simulink model "GFLI_full_standard"  (R2024b)
settings: Solver=FixedStepAuto  StartTime=0.0  StopTime=1  FixedStep=Ts  RelTol=1e-3
PreLoadFcn:
  | % Ts = 1e-6;
  | % Ts_Control = 50e-6;
  | %
  | % vlink = 700;
  | % Lf = 2.2e-3;
  | % Cf = 10e-6;
InitFcn:
  | clear all
  | clc
  | %% System parameters
  | Prated = 5e3; %5kW
  | Vg  = 220;     % rms grid voltage
  | Irms = Prated/(sqrt(3)*220*sqrt(3));
  | Ipk = Irms*sqrt(2);
  | 
  | Vdc = 700;     %dc-voltage
  | w1  = 100*pi;   % angular freq
  | fs  = 20e3;
  | Ts = 1/fs;      % control sampling time
  | fsw = 10e3;     % switching freq
  | Tsw = 1/fsw;
  | % grid param
  | Rg = 3e-4;
  | Lg = 1e-3;
  | %% LCL design
  | % Step A — pick inverter-side inductor L1 from ripple 20% Ipk
  | deltaI = 0.02*Ipk;
  | Lf1 = Vdc/(12*fsw*deltaI);
  | Rf1 = 3e-4;
  | % Step B — choose capacitor Cf by limiting reactive power at 50 Hz| Q =
  | %3*Vrms^2*w*Cf| limit ~3% => <= 150Var
  | Cf  = 150/(3*Vg^2*w1);
  | % Step C — choose grid-side inductor| L2/L1 ~ 0.3-1
  | Rf2 = 3e-4;
  | Lf2 = 1.5e-3;
  | % Step D — check resonance frequency|Rule of thumb: 10f1 < fr < 0.5fsw​
  | fr = (1/(2*pi))*sqrt((Lf1+Lf2)/(Lf1*Lf2*Cf));
  | wr = 2*pi*fr;
  | % Step E — damping: Passive damping resistor in series with Cf|
  | rd = 1/(3*wr*Cf);
  | 
  | %% PLL design| Bandwidth choice Typical 10–30 Hz. Choose 20 Hz:
  | wnPll = 2*pi*50;
  | xipll = 0.707;
  | Kp_pll = 2*xipll*wnPll;
  | Ki_pll = wnPll^2;
  | 
  | %% PI current controller|
  | Tresc=0.5e-3;
  | e=1;
  | omega=2*pi/Tresc;
  | k=1/(Lf1+Lf2);
  | Kp_PI=2*e*omega/k;
  | Ki_PI=omega^2/k;
undefined symbols (not defined in the file or in its folder): DiscIntNeverNeededParam, initial
libraries: spsVoltageMeasurementLib x13, spsCurrentMeasurementLib x6, spsIGBTDiodeLib x6, spsSeriesRLCBranchLib x6, powerlib_extras x4, spsThreePhaseSeriesRLCBranchLib x3, spsPLL3phLib x1, spsPWMGenerator2LevelLib x1, spsDCVoltageSourceLib x1, spsThreePhaseSourceLib x1, sps_lib x1
settings Model: Creator=hjyoo  LastModifiedBy=ACER
settings RTWCC: GPUComputeCapability=3.5

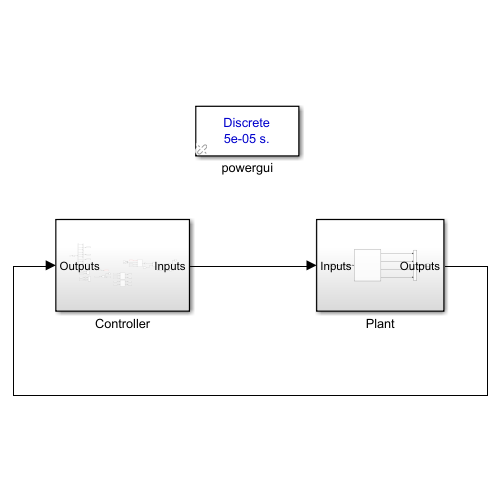
[thumbnail: Simulink's stored preview of the top-level diagram]
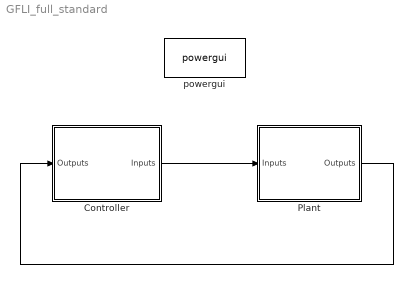
== system GFLI_full_standard ==
  Controller : Subsystem
  Plant : Subsystem
  powergui : sps_lib/powergui  Priority=1  SimulationMode=Discrete  SampleTime=Ts  frequency=60  Iterations=50  frequencyindice=0  Pbase=100e6  ErrMax=1e-4  UnitsV=kV  UnitsW=MW  buscounter=0  FunctionMessages=off  echomessages=off  EnableUseOfTLC=off  CurrentSourceSwitches=off  DisableSnubberDevices=off  DisableRonSwitches=off  DisableVfSwitches=off  DisplayEquations=off  AutomaticDiscreteSolvers=off  SolverType=Tustin/Backward Euler (TBE)  Interpol=off  ExternalGateDelay=off  methode=off  Ts=100  x0status=blocks  SPID=on  SwTol=0  HookPort=off  NonlinearTolerance=1e-4  nMaxIteration=100  ContinueOnMaxIteration=off  RestoreLinks=warning  ResistiveCurrentMeasurement=off  Frange=[0:2:500]  Ylog=off  Xlog=on  ShowGrid=off  save=off  variable=ZData  structure=0  ZoomFFT=off  StartTime=0.0  cycles=1  DisplayStyle=1  fundamental=60  FreqAxis=off  MaxFrequency=1000  frequencyindicesteady=1  RmsSteady=1  display=off
  wires:
  Controller/1(Inputs) -> Plant/1(Inputs)
  Plant/1(Outputs) -> Controller/1(Outputs)

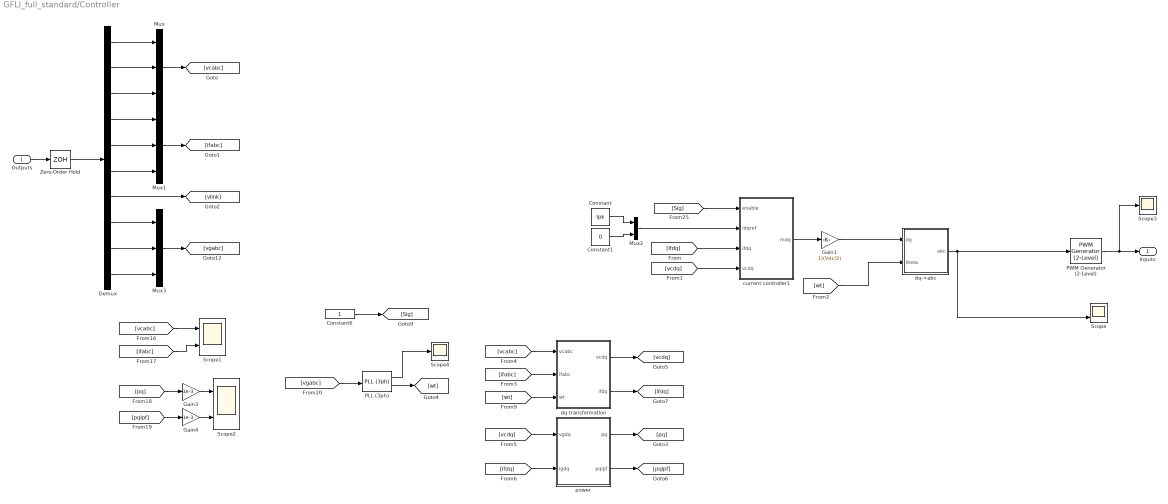
== system GFLI_full_standard/Controller ==
  Outputs : Inport
  Constant : Constant  Value=Ipk
  Constant1 : Constant  Value=0
  Constant6 : Constant
  Demux : Demux  Outputs=10
  Gain1 : Gain  Gain=1/(Vdc/2)
  Gain3 : Gain  Gain=1e-3
  Gain4 : Gain  Gain=1e-3
  Mux : Mux  Inputs=3
  Mux1 : Mux  Inputs=3
  Mux2 : Mux  Inputs=2
  Mux3 : Mux  Inputs=3
  PLL (3ph) : spsPLL3phLib/PLL (3ph)  Fmin=45  Par_Init=[0, 50]  ParK=[180, 3200, 1]  TcD=1e-4  MaxRateChangeFreq=12  FilterCutOffFreq=25  Ts=0  AGC=on
  PWM Generator (2-Level) : spsPWMGenerator2LevelLib/PWM Generator (2-Level)  ModulatorType=Three-phase bridge (6 pulses)  ModulatorMode=Unsynchronized  Fc=fsw  Pc=0  nF=27  MinMax="[ -1  1 ]"  SamplingTechnique=Natural  ModulatingSignals=off  m=0.8  Freq=60  Phase=0  Ts=Ts  ShowCarrierOutport=off
  Scope : Scope  NumInputPorts=2
  Scope1 : Scope  NumInputPorts=2
  Scope2 : Scope  NumInputPorts=2
  Scope3 : Scope
  Scope4 : Scope
  Zero-Order Hold : ZeroOrderHold  SampleTime=Ts
  current controller1 : Subsystem  mask{kp=Kp_PI, ki=Ki_PI, limit=inf, L=Lf1+Lf2, ts=Ts}
      mask prompts: kp "proportional(kp)"; ki "integral(ki)"; limit "saturation limit"; L "inductance(H)"; ts "Sampling Time"
  dq transformation : Subsystem
  dq->abc : Subsystem
  power : Subsystem
  Inputs : Outport
  wires:
  Outputs/1 -> Zero-Order Hold/1
  Demux/1 -> Mux/1
  Demux/2 -> Mux/2
  Demux/3 -> Mux/3
  Demux/5 -> Mux1/2
  Demux/4 -> Mux1/1
  Demux/6 -> Mux1/3
  Mux1/1 -> [ifabc]
  Demux/7 -> [vlink]
  Zero-Order Hold/1 -> Demux/1
  PWM Generator (2-Level)/1 -> Scope3/1, Inputs/1
  Mux/1 -> [vcabc]
  dq transformation/2(ifdq) -> [ifdq]
  dq transformation/1(vcdq) -> [vcdq]
  [vcabc] -> dq transformation/1(vcabc)
  [wt] -> dq transformation/3(wt)
  [ifabc] -> dq transformation/2(ifabc)
  [ifdq] -> current controller1/3(ifdq)
  [wt] -> dq->abc/2(theta)
  dq->abc/1(abc) -> Scope/2, PWM Generator (2-Level)/1
  [vcdq] -> power/1(vgdq)
  power/1(pq) -> [pq]
  [ifdq] -> power/2(igdq)
  power/2(pqlpf) -> [pqlpf]
  [vcdq] -> current controller1/4(vcdq)
  current controller1/1(mdq) -> Gain1/1
  [Sig] -> current controller1/1(enable)
  Constant6/1 -> [Sig]
  [vcabc] -> Scope1/1
  [ifabc] -> Scope1/2
  [pq] -> Gain3/1
  [pqlpf] -> Gain4/1
  Gain3/1 -> Scope2/1
  Gain4/1 -> Scope2/2
  Constant/1 -> Mux2/1
  Constant1/1 -> Mux2/2
  Mux2/1 -> current controller1/2(idqref)
  Mux3/1 -> [vgabc]
  Demux/10 -> Mux3/3
  Demux/8 -> Mux3/1
  Demux/9 -> Mux3/2
  [vgabc] -> PLL (3ph)/1
  PLL (3ph)/2 -> [wt]
  PLL (3ph)/1 -> Scope4/1
  Gain1/1 -> dq->abc/1(dq)

== system GFLI_full_standard/Plant ==
  Inputs : Inport
  Mux : Mux  Inputs=[3 3 1 3]
  Subsystem : Subsystem
  Outputs : Outport
  wires:
  Subsystem/2(ifabc) -> Mux/2
  Subsystem/3(vlink) -> Mux/3
  Mux/1 -> Outputs/1
  Subsystem/1(vcabc) -> Mux/1
  Inputs/1 -> Subsystem/1(PWM)
  Subsystem/4(vgabc) -> Mux/4

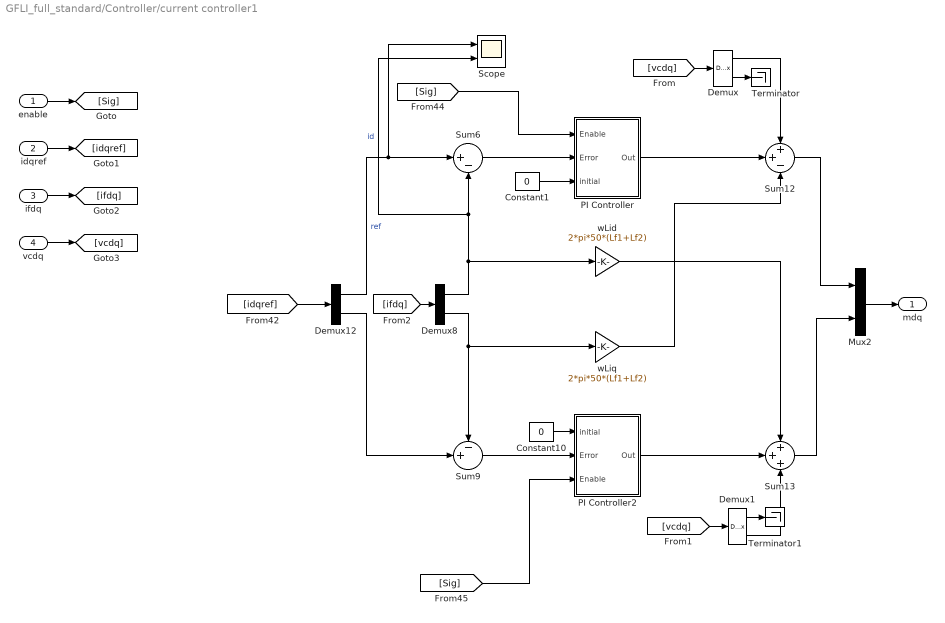
== system GFLI_full_standard/Controller/current controller1 ==
  enable : Inport
  idqref : Inport  Port=2
  ifdq : Inport  Port=3
  vcdq : Inport  Port=4
  Constant1 : Constant  Value=0
  Constant10 : Constant  Value=0
  Demux{,1,8,12} (4 alike) : Demux  Outputs=2
  Mux2 : Mux  Inputs=2
  PI Controller : Subsystem  mask{Kp=kp, Ki=ki, limit=limit, ts=ts}
      mask prompts: Kp "Proportional(Kp)"; Ki "Integral(Ki)"; limit "Saturation limit"; ts "Sampling Time"
  PI Controller2 : Subsystem  mask{Kp=kp, Ki=ki, limit=limit, ts=ts}
      mask prompts: Kp "Proportional(Kp)"; Ki "Integral(Ki)"; limit "Saturation limit"; ts "Sampling Time"
  Scope : Scope  NumInputPorts=2
  Sum12 : Sum  Inputs=++-
  Sum13 : Sum  Inputs=+++
  Sum6 : Sum  Inputs=|+-
  Sum9 : Sum  Inputs=-+|
  Terminator : Terminator
  Terminator1 : Terminator
  wLid : Gain  Gain=2*pi*50*(Lf1+Lf2)
  wLiq : Gain  Gain=2*pi*50*(Lf1+Lf2)
  mdq : Outport  VectorParamsAs1DForOutWhenUnconnected=off
  wires:
  PI Controller2/1(Out) -> Sum13/2
  [idqref] -> Demux12/1
  Sum6/1 -> PI Controller/2(Error)
  Demux8/2 -> Sum9/1, wLiq/1
  Sum12/1 -> Mux2/1
  wLiq/1 -> Sum12/3
  [Sig] -> PI Controller/1(Enable)
  PI Controller/1(Out) -> Sum12/2
  Sum9/1 -> PI Controller2/2(Error)
  Demux8/1 -> Scope/2, Sum6/2, wLid/1  "id"
  Demux12/2 -> Sum9/2
  Demux12/1 -> Scope/1, Sum6/1  "ref"
  wLid/1 -> Sum13/1
  [ifdq] -> Demux8/1
  Sum13/1 -> Mux2/2
  enable/1 -> [Sig]
  idqref/1 -> [idqref]
  ifdq/1 -> [ifdq]
  vcdq/1 -> [vcdq]
  Mux2/1 -> mdq/1
  Constant10/1 -> PI Controller2/1(initial)
  [Sig] -> PI Controller2/3(Enable)
  Constant1/1 -> PI Controller/3(initial)
  [vcdq] -> Demux/1
  Demux/1 -> Sum12/1
  [vcdq] -> Demux1/1
  Demux1/2 -> Sum13/3
  Demux/2 -> Terminator/1
  Demux1/1 -> Terminator1/1

== system GFLI_full_standard/Controller/dq transformation ==
  vcabc : Inport
  ifabc : Inport  Port=2
  wt : Inport  Port=3
  Selector : Selector  InputPortWidth=3  IndexOptions=Index vector (dialog)  Indices=[1 2 ]  OutputSizes=1
  Selector1 : Selector  InputPortWidth=3  IndexOptions=Index vector (dialog)  Indices=[1 2]  OutputSizes=1
  Subsystem3 : Subsystem
  Subsystem4 : Subsystem
  abc_to_dq0 Transformation : powerlib_extras/Measurements/abc_to_dq0 Transformation
  abc_to_dq0 Transformation1 : powerlib_extras/Measurements/abc_to_dq0 Transformation
  vcdq : Outport
  ifdq : Outport  Port=2
  wires:
  wt/1 -> Subsystem3/1(wt), Subsystem4/1(wt)
  Selector/1 -> vcdq/1
  ifabc/1 -> abc_to_dq0 Transformation1/1
  Selector1/1 -> ifdq/1
  vcabc/1 -> abc_to_dq0 Transformation/1
  abc_to_dq0 Transformation/1 -> Selector/1
  abc_to_dq0 Transformation1/1 -> Selector1/1
  Subsystem4/1(s_c) -> abc_to_dq0 Transformation1/2
  Subsystem3/1(s_c) -> abc_to_dq0 Transformation/2

== system GFLI_full_standard/Controller/dq->abc ==
  dq : Inport
  theta : Inport  Port=2
  Mux1 : Mux  Inputs=2
  Mux2 : Mux  Inputs=3
  dq->a : Fcn  Expr=u[1]*sin(u[3])+u[2]*cos(u[3])
  dq->b : Fcn  Expr=u[1]*sin(u[3]-(2*pi/3))+u[2]*cos(u[3]-(2*pi/3))
  dq->c : Fcn  Expr=u[1]*sin(u[3]+(2*pi/3))+u[2]*cos(u[3]+(2*pi/3))
  abc : Outport
  wires:
  Mux1/1 -> dq->a/1, dq->b/1, dq->c/1
  dq->b/1 -> Mux2/2
  dq->c/1 -> Mux2/3
  dq->a/1 -> Mux2/1
  Mux2/1 -> abc/1
  dq/1 -> Mux1/1
  theta/1 -> Mux1/2

== system GFLI_full_standard/Controller/power ==
  vgdq : Inport
  igdq : Inport  Port=2
  LPF : Subsystem  mask{Fc=20}
      mask prompts: Fc "Cut off frequency"
  Mux3 : Mux  Inputs=[2 2]
  Mux5 : Mux  Inputs=2
  p : Fcn  Expr=1.5*((u(1)*u(3)) + (u(2)*u(4)))
  q : Fcn  Expr=1.5*((u(2)*u(3)) - (u(1)*u(4)))
  pq : Outport
  pqlpf : Outport  Port=2
  wires:
  igdq/1 -> Mux3/2
  q/1 -> Mux5/2
  Mux3/1 -> p/1, q/1
  vgdq/1 -> Mux3/1
  p/1 -> Mux5/1
  Mux5/1 -> pq/1, LPF/1(In1)
  LPF/1(Out1) -> pqlpf/1

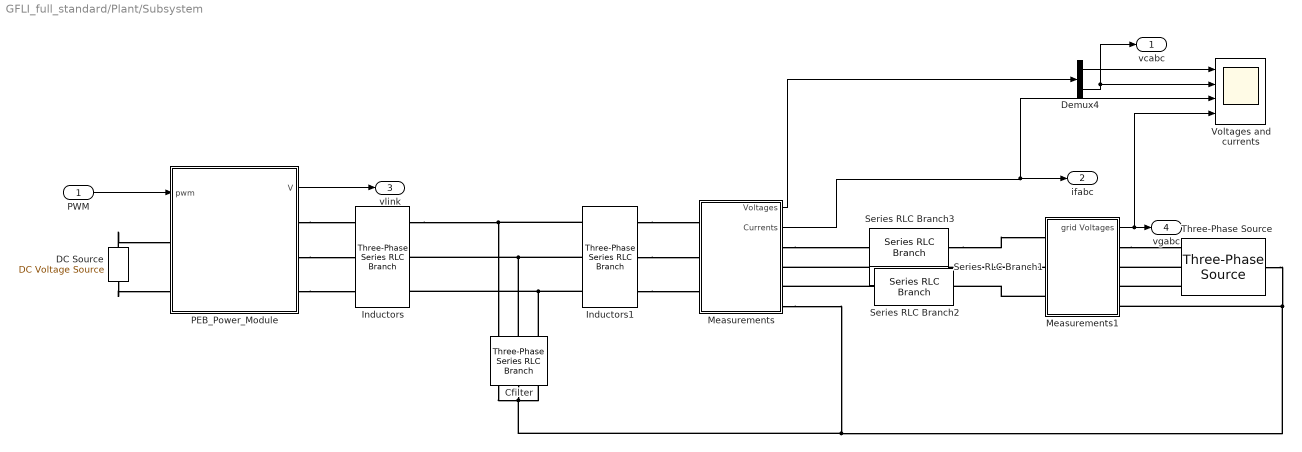
== system GFLI_full_standard/Plant/Subsystem ==
  PWM : Inport
  Cfilter : spsThreePhaseSeriesRLCBranchLib/Three-Phase Series RLC Branch  LConnTagsString=A|B|C  RConnTagsString=A|B|C  BranchType=RC  Resistance=rd  Inductance=2.2e-3  Capacitance=Cf  Measurements=None
  DC Source : spsDCVoltageSourceLib/DC Voltage Source  Amplitude=Vdc  Measurements=None
  Demux4 : Demux  Outputs=[3 3]
  Inductors : spsThreePhaseSeriesRLCBranchLib/Three-Phase Series RLC Branch  LConnTagsString=A|B|C  RConnTagsString=A|B|C  BranchType=RL  Resistance=Rf1  Inductance=Lf1  Capacitance=1e-6  Measurements=None
  Inductors1 : spsThreePhaseSeriesRLCBranchLib/Three-Phase Series RLC Branch  LConnTagsString=A|B|C  RConnTagsString=A|B|C  BranchType=RL  Resistance=Rf2  Inductance=Lf2  Capacitance=1e-6  Measurements=None
  Measurements : Subsystem
  Measurements1 : Subsystem
  PEB_Power_Module : Subsystem
  Series RLC Branch1 : spsSeriesRLCBranchLib/Series RLC Branch  LConnTagsString=__new0  RConnTagsString=__new0  BranchType=RL  Resistance=Rg  Inductance=Lg  SetiL0=off  InitialCurrent=0  Capacitance=1e-6  Setx0=off  InitialVoltage=0  Measurements=None
  Series RLC Branch2 : spsSeriesRLCBranchLib/Series RLC Branch  LConnTagsString=__new0  RConnTagsString=__new0  BranchType=RL  Resistance=Rg  Inductance=Lg  SetiL0=off  InitialCurrent=0  Capacitance=1e-6  Setx0=off  InitialVoltage=0  Measurements=None
  Series RLC Branch3 : spsSeriesRLCBranchLib/Series RLC Branch  LConnTagsString=__new0  RConnTagsString=__new0  BranchType=RL  Resistance=Rg  Inductance=Lg  SetiL0=off  InitialCurrent=0  Capacitance=1e-6  Setx0=off  InitialVoltage=0  Measurements=None
  Three-Phase Source : spsThreePhaseSourceLib/Three-Phase Source  InternalConnection=Yn  VoltagePhases=off  Voltage=Vg*sqrt(3)  PhaseAngle=0  Voltage_phases=[25e3 25e3 25e3]/sqrt(3)  PhaseAngles_phases=[0 -120 +120]  Frequency=50  NonIdealSource=off  SpecifyImpedance=off  Resistance=0.8929  Inductance=16.58e-3  ShortCircuitLevel=100e6  BaseVoltage=25e3  XRratio=7  BusType=swing  Pref=10e3  Qref=0  Prefabc=[10e3, 10e3, 10e3]  Qrefabc=[0, 0, 0]  Qmin=-inf  Qmax=inf
  Voltages and currents : Scope  NumInputPorts=4
  vcabc : Outport
  ifabc : Outport  Port=2
  vlink : Outport  Port=3
  vgabc : Outport  Port=4
  wires:
  Demux4/2 -> vcabc/1, Voltages and currents/2
  Demux4/1 -> Voltages and currents/1
  PWM/1 -> PEB_Power_Module/1(pwm)
  Measurements/1(Voltages) -> Demux4/1
  Measurements/2(Currents) -> Voltages and currents/3, ifabc/1
  PEB_Power_Module/1(V) -> vlink/1
  Measurements1/1(grid Voltages) -> Voltages and currents/4, vgabc/1
  connections:
  Cfilter/LConn2 -- Inductors/RConn2 -- Inductors1/LConn2
  Cfilter/LConn3 -- Inductors/RConn3 -- Inductors1/LConn3
  Inductors/RConn1 -- Inductors1/LConn1 -- Cfilter/LConn1
  PEB_Power_Module/RConn1 -- Inductors/LConn1
  PEB_Power_Module/RConn2 -- Inductors/LConn2
  PEB_Power_Module/RConn3 -- Inductors/LConn3
  DC Source/RConn1 -- PEB_Power_Module/LConn1
  DC Source/LConn1 -- PEB_Power_Module/LConn2
  Series RLC Branch2/LConn1 -- Measurements/RConn3
  Measurements/RConn1 -- Series RLC Branch3/LConn1
  Series RLC Branch1/LConn1 -- Measurements/RConn2
  Inductors1/RConn1 -- Measurements/LConn1
  Inductors1/RConn3 -- Measurements/LConn3
  Inductors1/RConn2 -- Measurements/LConn2
  Measurements/RConn4 -- Measurements1/RConn4 -- Three-Phase Source/LConn1 -- Cfilter/RConn1 -- Cfilter/RConn2 -- Cfilter/RConn3
  Three-Phase Source/RConn1 -- Measurements1/RConn3
  Measurements1/LConn3 -- Series RLC Branch2/RConn1
  Measurements1/LConn2 -- Series RLC Branch1/RConn1
  Series RLC Branch3/RConn1 -- Measurements1/LConn1
  Three-Phase Source/RConn2 -- Measurements1/RConn2
  Measurements1/RConn1 -- Three-Phase Source/RConn3

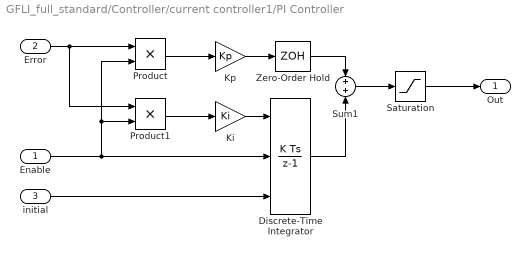
== system GFLI_full_standard/Controller/current controller1/PI Controller ==
  Enable : Inport
  Error : Inport  Port=2
  initial : Inport  Port=3
  Discrete-Time Integrator : DiscreteIntegrator  gainval=1  ExternalReset=rising  InitialConditionSource=external  InitialCondition=initial  SampleTime=ts  LimitOutput=on  UpperSaturationLimit=limit  LowerSaturationLimit=-limit  ICPrevOutput=DiscIntNeverNeededParam  ICPrevScaledInput=DiscIntNeverNeededParam
  Ki : Gain  Gain=Ki  SaturateOnIntegerOverflow=on  OutDataTypeStr=Inherit: Same as input  ParamDataTypeStr=Inherit: Same as input
  Kp : Gain  Gain=Kp  SaturateOnIntegerOverflow=on  OutDataTypeStr=Inherit: Same as input  ParamDataTypeStr=Inherit: Same as input
  Product : Product
  Product1 : Product
  Saturation : Saturate  UpperLimit=limit  LowerLimit=-limit
  Sum1 : Sum  SaturateOnIntegerOverflow=on
  Zero-Order Hold : ZeroOrderHold  SampleTime=Ts
  Out : Outport
  wires:
  Ki/1 -> Discrete-Time Integrator/1
  initial/1 -> Discrete-Time Integrator/3
  Saturation/1 -> Out/1
  Enable/1 -> Discrete-Time Integrator/2, Product/2, Product1/2
  Sum1/1 -> Saturation/1
  Kp/1 -> Zero-Order Hold/1
  Discrete-Time Integrator/1 -> Sum1/2
  Product/1 -> Kp/1
  Product1/1 -> Ki/1
  Error/1 -> Product1/1, Product/1
  Zero-Order Hold/1 -> Sum1/1

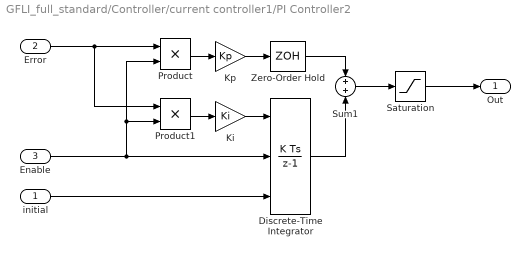
== system GFLI_full_standard/Controller/current controller1/PI Controller2 ==
  initial : Inport
  Error : Inport  Port=2
  Enable : Inport  Port=3
  Discrete-Time Integrator : DiscreteIntegrator  gainval=1  ExternalReset=rising  InitialConditionSource=external  InitialCondition=initial  SampleTime=ts  LimitOutput=on  UpperSaturationLimit=limit  LowerSaturationLimit=-limit  ICPrevOutput=DiscIntNeverNeededParam  ICPrevScaledInput=DiscIntNeverNeededParam
  Ki : Gain  Gain=Ki  SaturateOnIntegerOverflow=on  OutDataTypeStr=Inherit: Same as input  ParamDataTypeStr=Inherit: Same as input
  Kp : Gain  Gain=Kp  SaturateOnIntegerOverflow=on  OutDataTypeStr=Inherit: Same as input  ParamDataTypeStr=Inherit: Same as input
  Product : Product
  Product1 : Product
  Saturation : Saturate  UpperLimit=limit  LowerLimit=-limit
  Sum1 : Sum  SaturateOnIntegerOverflow=on
  Zero-Order Hold : ZeroOrderHold  SampleTime=Ts
  Out : Outport
  wires:
  Error/1 -> Product/1, Product1/1
  Product1/1 -> Ki/1
  Product/1 -> Kp/1
  Discrete-Time Integrator/1 -> Sum1/2
  Kp/1 -> Zero-Order Hold/1
  Sum1/1 -> Saturation/1
  Enable/1 -> Discrete-Time Integrator/2, Product1/2, Product/2
  Saturation/1 -> Out/1
  initial/1 -> Discrete-Time Integrator/3
  Ki/1 -> Discrete-Time Integrator/1
  Zero-Order Hold/1 -> Sum1/1

== system GFLI_full_standard/Controller/dq transformation/Subsystem3 ==
  wt : Inport
  Mux2 : Mux  Inputs=2
  Trigonometric Function1 : Trigonometry
  Trigonometric Function3 : Trigonometry  Operator=cos
  s_c : Outport
  wires:
  Mux2/1 -> s_c/1
  Trigonometric Function1/1 -> Mux2/1
  Trigonometric Function3/1 -> Mux2/2
  wt/1 -> Trigonometric Function1/1, Trigonometric Function3/1

== system GFLI_full_standard/Controller/dq transformation/Subsystem4 ==
  wt : Inport
  Mux2 : Mux  Inputs=2
  Trigonometric Function1 : Trigonometry
  Trigonometric Function3 : Trigonometry  Operator=cos
  s_c : Outport
  wires:
  wt/1 -> Trigonometric Function3/1, Trigonometric Function1/1
  Trigonometric Function3/1 -> Mux2/2
  Trigonometric Function1/1 -> Mux2/1
  Mux2/1 -> s_c/1

== system GFLI_full_standard/Controller/power/LPF ==
  In1 : Inport
  Demux8 : Demux  Outputs=2
  Discrete 2nd-Order Filter1 : powerlib_extras/Discrete  Control Blocks/Discrete  2nd-Order Filter  FilterType=Lowpass  Fo=Fc  Zeta=0.707  Ts=Ts  Initialize=off  Vac_Init=[0.8 -25 60]  Vdc_Init=-0.4  PlotResponse=off  param1=[1 500 1]
  Discrete 2nd-Order Filter2 : powerlib_extras/Discrete  Control Blocks/Discrete  2nd-Order Filter  FilterType=Lowpass  Fo=Fc  Zeta=0.707  Ts=Ts  Initialize=off  Vac_Init=[0.8 -25 60]  Vdc_Init=-0.4  PlotResponse=off  param1=[1 500 1]
  Mux4 : Mux  Inputs=2
  Out1 : Outport
  wires:
  Demux8/1 -> Discrete 2nd-Order Filter2/1
  Demux8/2 -> Discrete 2nd-Order Filter1/1
  Discrete 2nd-Order Filter2/1 -> Mux4/1
  Discrete 2nd-Order Filter1/1 -> Mux4/2
  In1/1 -> Demux8/1
  Mux4/1 -> Out1/1

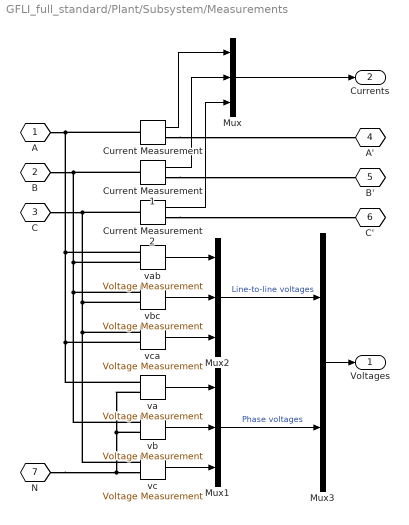
== system GFLI_full_standard/Plant/Subsystem/Measurements ==
  Current Measurement : spsCurrentMeasurementLib/Current Measurement  PhasorSimulation=off  OutputType=Complex  PSBequivalent=0
  Current Measurement1 : spsCurrentMeasurementLib/Current Measurement  PhasorSimulation=off  OutputType=Complex  PSBequivalent=0
  Current Measurement2 : spsCurrentMeasurementLib/Current Measurement  PhasorSimulation=off  OutputType=Complex  PSBequivalent=0
  Mux : Mux  Inputs=3
  Mux1 : Mux  Inputs=3
  Mux2 : Mux  Inputs=3
  Mux3 : Mux  Inputs=[3 3]
  va : spsVoltageMeasurementLib/Voltage Measurement  PhasorSimulation=off  OutputType=Complex  PSBequivalent=0
  vab : spsVoltageMeasurementLib/Voltage Measurement  PhasorSimulation=off  OutputType=Complex  PSBequivalent=0
  vb : spsVoltageMeasurementLib/Voltage Measurement  PhasorSimulation=off  OutputType=Complex  PSBequivalent=0
  vbc : spsVoltageMeasurementLib/Voltage Measurement  PhasorSimulation=off  OutputType=Complex  PSBequivalent=0
  vc : spsVoltageMeasurementLib/Voltage Measurement  PhasorSimulation=off  OutputType=Complex  PSBequivalent=0
  vca : spsVoltageMeasurementLib/Voltage Measurement  PhasorSimulation=off  OutputType=Complex  PSBequivalent=0
  A : PMIOPort  Tag=PMCPort  Side=Left
  B : PMIOPort  Tag=PMCPort  Port=2  Side=Left
  C : PMIOPort  Tag=PMCPort  Port=3  Side=Left
  A' : PMIOPort  Tag=PMCPort  Port=4  Side=Right
  B' : PMIOPort  Tag=PMCPort  Port=5  Side=Right
  C' : PMIOPort  Tag=PMCPort  Port=6  Side=Right
  N : PMIOPort  Tag=PMCPort  Port=7  Side=Right
  Voltages : Outport
  Currents : Outport  Port=2
  wires:
  Current Measurement/1 -> Mux/1
  Current Measurement1/1 -> Mux/2
  Current Measurement2/1 -> Mux/3
  Mux/1 -> Currents/1
  vb/1 -> Mux1/2
  va/1 -> Mux1/1
  vc/1 -> Mux1/3
  vab/1 -> Mux2/1
  vbc/1 -> Mux2/2
  vca/1 -> Mux2/3
  Mux3/1 -> Voltages/1
  Mux1/1 -> Mux3/2  "Phase voltages"
  Mux2/1 -> Mux3/1  "Line-to-line voltages"
  connections:
  B/RConn1 -- Current Measurement1/LConn1 -- vab/LConn2 -- vbc/LConn1 -- vb/LConn1
  vab/LConn1 -- vca/LConn2 -- va/LConn1 -- Current Measurement/LConn1 -- A/RConn1
  C/RConn1 -- Current Measurement2/LConn1 -- vbc/LConn2 -- vca/LConn1 -- vc/LConn1
  Current Measurement2/RConn1 -- C'/RConn1
  Current Measurement1/RConn1 -- B'/RConn1
  Current Measurement/RConn1 -- A'/RConn1
  N/RConn1 -- vb/LConn2 -- va/LConn2 -- vc/LConn2

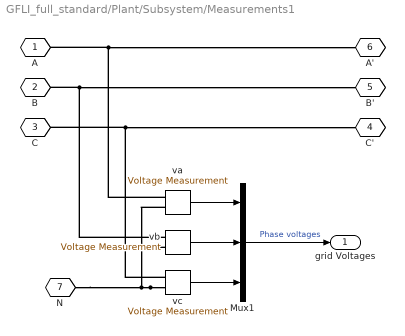
== system GFLI_full_standard/Plant/Subsystem/Measurements1 ==
  Mux1 : Mux  Inputs=3
  va : spsVoltageMeasurementLib/Voltage Measurement  PhasorSimulation=off  OutputType=Complex  PSBequivalent=0
  vb : spsVoltageMeasurementLib/Voltage Measurement  PhasorSimulation=off  OutputType=Complex  PSBequivalent=0
  vc : spsVoltageMeasurementLib/Voltage Measurement  PhasorSimulation=off  OutputType=Complex  PSBequivalent=0
  A : PMIOPort  Tag=PMCPort  Side=Left
  B : PMIOPort  Tag=PMCPort  Port=2  Side=Left
  C : PMIOPort  Tag=PMCPort  Port=3  Side=Left
  C' : PMIOPort  Tag=PMCPort  Port=4  Side=Right
  B' : PMIOPort  Tag=PMCPort  Port=5  Side=Right
  A' : PMIOPort  Tag=PMCPort  Port=6  Side=Right
  N : PMIOPort  Tag=PMCPort  Port=7  Side=Right
  grid Voltages : Outport
  wires:
  Mux1/1 -> grid Voltages/1  "Phase voltages"
  vc/1 -> Mux1/3
  va/1 -> Mux1/1
  vb/1 -> Mux1/2
  connections:
  vc/LConn2 -- va/LConn2 -- vb/LConn2 -- N/RConn1
  va/LConn1 -- A/RConn1 -- A'/RConn1
  vb/LConn1 -- B'/RConn1 -- B/RConn1
  vc/LConn1 -- C'/RConn1 -- C/RConn1

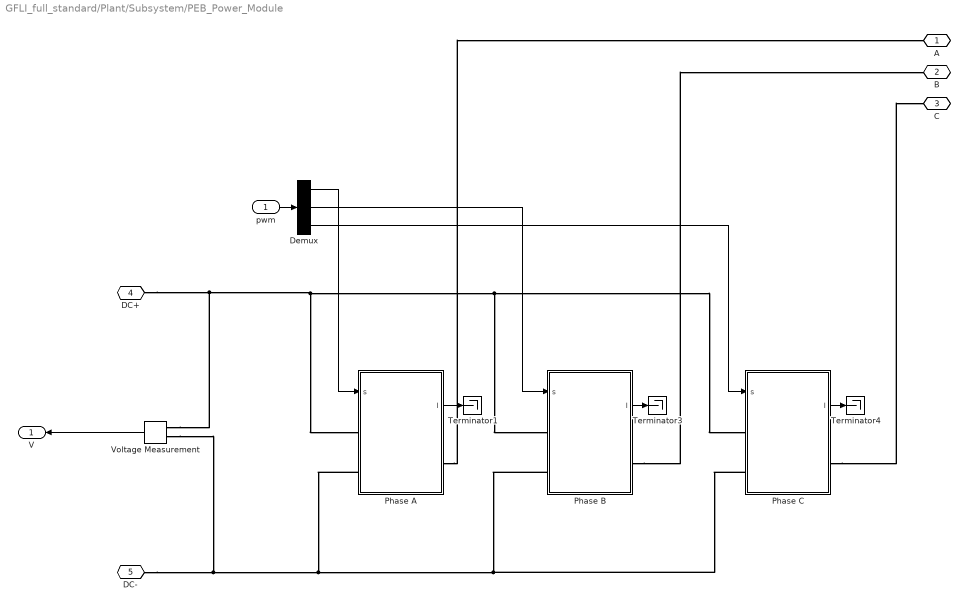
== system GFLI_full_standard/Plant/Subsystem/PEB_Power_Module ==
  pwm : Inport
  Demux : Demux  Outputs=[2 2 2]
  Phase A : Subsystem  mask{pV0=Vdc, pOutputCurrent=on, pOutputVoltage=off}
      mask prompts: pV0 "Initial DC bus voltage"; pOutputCurrent "Show current measurement output"; pOutputVoltage "Show voltage measurement output"
      mask init:
      | % show/hide current measurement port
      | if strcmp(get_param(gcb, 'pOutputCurrent'), 'on')
      |     if strcmp(get_param([gcb,'/I'],'BlockType'),'Terminator')
      |         temp = get_param([gcb,'/I'],'position');
      |         delete_block([gcb,'/I']);
      |         add_block('built-in/Outport',[gcb,'/I']);
      |         set_param([gcb,'/I'],'position',temp);
      |     end
      | else
      |     if strcmp(get_param([gcb,'/I'],'BlockType'),'Outport')
      |         temp = get_param([gcb,'/I'],'position');
      |         delete_block([gcb,'/I']);
      |         add_block('built-in/Terminator',[gcb,'/I']);
      |         set_param([gcb,'/I'],'position',temp);
      |     end
      | end
      | 
      | % show/hide volatge measurement port
      | if strcmp(get_param(gcb, 'pOutputVoltage'), 'on')
      |     if strcmp(get_param([gcb,'/V'],'BlockType'),'Terminator')
      |         temp = get_param([gcb,'/V'],'position');
      |         delete_block([gcb,'/V']);
      |         add_block('built-in/Outport',[gcb,'/V']);
      |         set_param([gcb,'/V'],'position',temp);
      |     end
      | else
      |     if strcmp(get_param([gcb,'/V'],'BlockType'),'Outport')
      |         temp = get_param([gcb,'/V'],'position');
      |         delete_block([gcb,'/V']);
      |         add_block('built-in/Terminator',[gcb,'/V']);
      |         set_param([gcb,'/V'],'position',temp);
      |     end
      | end
      mask Display:
      | x1=0.0;
      | plot([0.15 0.5]+x1,[0.95 0.95])
      | plot([0.5 0.5]+x1,[0.95,0.80])
      | plot([0.5 0.38]+x1,[0.80 0.74])
      | plot([0.38 0.38]+x1,[0.80 0.62])
      | plot([0.38 0.5]+x1,[0.68 0.62])
      | plot([0.5 0.5]+x1,[0.62 0.52])
      | plot([0.45 0.5 0.43]+x1,[0.68 0.62 0.60])
      | %
      | y1=0.40;
      | plot([0.5 0.5]+x1,[0.95,0.80]-y1)
      | plot([0.5 0.38]+x1,[0.80 0.74]-y1)
      | plot([0.38 0.38]+x1,[0.80 0.62]-y1)
      | plot([0.38 0.5]+x1,[0.68 0.62]-y1)
      | plot([0.5 0.5]+x1,[0.62 0.52]-y1)
      | plot([0.45 0.5 0.43]+x1,[0.68 0.62 0.60]-y1)
      | plot([0.5 0.5]+x1,[0.2,0.10])
      | plot([0.15 0.5]+x1,[0.1 0.1])
      | %
      | plot([0.5 0.6]+x1,[0.84 0.84])
      | plot([0.6 0.6]+x1,[0.84 0.74])
      | plot([0.6 0.56]+x1,[0.74 0.69])
      | plot([0.6 0.64]+x1,[0.74 0.69])
      | plot([0.56 0.64]+x1,[0.69 0.69])
      | plot([0.6 0.6]+x1,[0.69 0.57])
      | plot([0.5 0.6]+x1,[0.57 0.57])
      | plot([0.55 0.65]+x1,[0.74 0.74])
      | %
      | y2=0.4;
      | plot([0.5 0.6]+x1,[0.84 0.84]-y2)
      | plot([0.6 0.6]+x1,[0.84 0.74]-y2)
      | plot([0.6 0.56]+x1,[0.74 0.69]-y2)
      | plot([0.6 0.64]+x1,[0.74 0.69]-y2)
      | plot([0.56 0.64]+x1,[0.69 0.69]-y2)
      | plot([0.6 0.6]+x1,[0.69 0.57]-y2)
      | plot([0.5 0.6]+x1,[0.57 0.57]-y2)
      | plot([0.55 0.65]+x1,[0.74 0.74]-y2)
      | %
      | plot([0.5 0.77]+x1,[0.5 0.5])
      | %
      | plot([0.34 0.34]+x1,[0.65 0.75])
      | plot([0.28 0.34]+x1,[0.7 0.7])
      | %
      | plot([0.34 0.34]+x1,[0.65 0.75]-y2)
      | plot([0.28 0.34]+x1,[0.7 0.7]-y2)
  Phase B : Subsystem  mask{pV0=Vdc, pOutputCurrent=on, pOutputVoltage=off}
      mask prompts: pV0 "Initial DC bus voltage"; pOutputCurrent "Show current measurement output"; pOutputVoltage "Show voltage measurement output"
      mask init: same as GFLI_full_standard/Plant/Subsystem/PEB_Power_Module/Phase A
      mask Display:
      | x1=0.0;
      | plot([0.15 0.5]+x1,[0.95 0.95])
      | plot([0.5 0.5]+x1,[0.95,0.80])
      | plot([0.5 0.38]+x1,[0.80 0.74])
      | plot([0.38 0.38]+x1,[0.80 0.62])
      | plot([0.38 0.5]+x1,[0.68 0.62])
      | plot([0.5 0.5]+x1,[0.62 0.52])
      | plot([0.45 0.5 0.43]+x1,[0.68 0.62 0.60])
      | %
      | y1=0.40;
      | plot([0.5 0.5]+x1,[0.95,0.80]-y1)
      | plot([0.5 0.38]+x1,[0.80 0.74]-y1)
      | plot([0.38 0.38]+x1,[0.80 0.62]-y1)
      | plot([0.38 0.5]+x1,[0.68 0.62]-y1)
      | plot([0.5 0.5]+x1,[0.62 0.52]-y1)
      | plot([0.45 0.5 0.43]+x1,[0.68 0.62 0.60]-y1)
      | plot([0.5 0.5]+x1,[0.2,0.10])
      | plot([0.15 0.5]+x1,[0.1 0.1])
      | %
      | plot([0.5 0.6]+x1,[0.84 0.84])
      | plot([0.6 0.6]+x1,[0.84 0.74])
      | plot([0.6 0.56]+x1,[0.74 0.69])
      | plot([0.6 0.64]+x1,[0.74 0.69])
      | plot([0.56 0.64]+x1,[0.69 0.69])
      | plot([0.6 0.6]+x1,[0.69 0.57])
      | plot([0.5 0.6]+x1,[0.57 0.57])
      | plot([0.55 0.65]+x1,[0.74 0.74])
      | %
      | y2=0.4;
      | plot([0.5 0.6]+x1,[0.84 0.84]-y2)
      | plot([0.6 0.6]+x1,[0.84 0.74]-y2)
      | plot([0.6 0.56]+x1,[0.74 0.69]-y2)
      | plot([0.6 0.64]+x1,[0.74 0.69]-y2)
      | plot([0.56 0.64]+x1,[0.69 0.69]-y2)
      | plot([0.6 0.6]+x1,[0.69 0.57]-y2)
      | plot([0.5 0.6]+x1,[0.57 0.57]-y2)
      | plot([0.55 0.65]+x1,[0.74 0.74]-y2)
      | %
      | plot([0.5 0.77]+x1,[0.5 0.5])
      | %
      | plot([0.34 0.34]+x1,[0.65 0.75])
      | plot([0.28 0.34]+x1,[0.7 0.7])
      | %
      | plot([0.34 0.34]+x1,[0.65 0.75]-y2)
      | plot([0.28 0.34]+x1,[0.7 0.7]-y2)
  Phase C : Subsystem  mask{pV0=Vdc, pOutputCurrent=on, pOutputVoltage=off}
      mask prompts: pV0 "Initial DC bus voltage"; pOutputCurrent "Show current measurement output"; pOutputVoltage "Show voltage measurement output"
      mask init: same as GFLI_full_standard/Plant/Subsystem/PEB_Power_Module/Phase A
      mask Display:
      | x1=0.0;
      | plot([0.15 0.5]+x1,[0.95 0.95])
      | plot([0.5 0.5]+x1,[0.95,0.80])
      | plot([0.5 0.38]+x1,[0.80 0.74])
      | plot([0.38 0.38]+x1,[0.80 0.62])
      | plot([0.38 0.5]+x1,[0.68 0.62])
      | plot([0.5 0.5]+x1,[0.62 0.52])
      | plot([0.45 0.5 0.43]+x1,[0.68 0.62 0.60])
      | %
      | y1=0.40;
      | plot([0.5 0.5]+x1,[0.95,0.80]-y1)
      | plot([0.5 0.38]+x1,[0.80 0.74]-y1)
      | plot([0.38 0.38]+x1,[0.80 0.62]-y1)
      | plot([0.38 0.5]+x1,[0.68 0.62]-y1)
      | plot([0.5 0.5]+x1,[0.62 0.52]-y1)
      | plot([0.45 0.5 0.43]+x1,[0.68 0.62 0.60]-y1)
      | plot([0.5 0.5]+x1,[0.2,0.10])
      | plot([0.15 0.5]+x1,[0.1 0.1])
      | %
      | plot([0.5 0.6]+x1,[0.84 0.84])
      | plot([0.6 0.6]+x1,[0.84 0.74])
      | plot([0.6 0.56]+x1,[0.74 0.69])
      | plot([0.6 0.64]+x1,[0.74 0.69])
      | plot([0.56 0.64]+x1,[0.69 0.69])
      | plot([0.6 0.6]+x1,[0.69 0.57])
      | plot([0.5 0.6]+x1,[0.57 0.57])
      | plot([0.55 0.65]+x1,[0.74 0.74])
      | %
      | y2=0.4;
      | plot([0.5 0.6]+x1,[0.84 0.84]-y2)
      | plot([0.6 0.6]+x1,[0.84 0.74]-y2)
      | plot([0.6 0.56]+x1,[0.74 0.69]-y2)
      | plot([0.6 0.64]+x1,[0.74 0.69]-y2)
      | plot([0.56 0.64]+x1,[0.69 0.69]-y2)
      | plot([0.6 0.6]+x1,[0.69 0.57]-y2)
      | plot([0.5 0.6]+x1,[0.57 0.57]-y2)
      | plot([0.55 0.65]+x1,[0.74 0.74]-y2)
      | %
      | plot([0.5 0.77]+x1,[0.5 0.5])
      | %
      | plot([0.34 0.34]+x1,[0.65 0.75])
      | plot([0.28 0.34]+x1,[0.7 0.7])
      | %
      | plot([0.34 0.34]+x1,[0.65 0.75]-y2)
      | plot([0.28 0.34]+x1,[0.7 0.7]-y2)
  Terminator1 : Terminator
  Terminator3 : Terminator
  Terminator4 : Terminator
  Voltage Measurement : spsVoltageMeasurementLib/Voltage Measurement  PhasorSimulation=off  OutputType=Complex  PSBequivalent=0
  A : PMIOPort  Side=Right
  B : PMIOPort  Port=2  Side=Right
  C : PMIOPort  Port=3  Side=Right
  DC+ : PMIOPort  Port=4  Side=Left
  DC- : PMIOPort  Port=5  Side=Left
  V : Outport
  wires:
  Phase C/1(I) -> Terminator4/1
  Phase B/1(I) -> Terminator3/1
  Demux/3 -> Phase C/1(s)
  Demux/2 -> Phase B/1(s)
  Demux/1 -> Phase A/1(s)
  pwm/1 -> Demux/1
  Phase A/1(I) -> Terminator1/1
  Voltage Measurement/1 -> V/1
  connections:
  DC+/RConn1 -- Voltage Measurement/LConn1 -- Phase A/LConn1 -- Phase C/LConn1 -- Phase B/LConn1
  DC-/RConn1 -- Voltage Measurement/LConn2 -- Phase A/LConn2 -- Phase C/LConn2 -- Phase B/LConn2
  Phase C/RConn1 -- C/RConn1
  Phase B/RConn1 -- B/RConn1
  Phase A/RConn1 -- A/RConn1

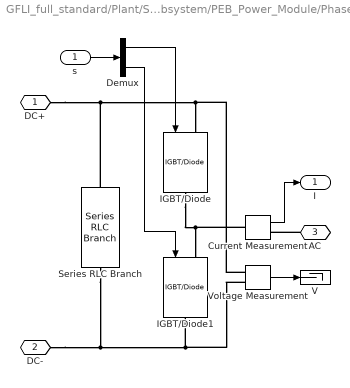
== system GFLI_full_standard/Plant/Subsystem/PEB_Power_Module/Phase A ==
  s : Inport
  Current Measurement : spsCurrentMeasurementLib/Current Measurement  PhasorSimulation=off  OutputType=Complex  PSBequivalent=0
  Demux : Demux  Outputs=2
  IGBT/Diode : spsIGBTDiodeLib/IGBT//Diode  Ron=1e-3  Rs=1e5  Cs=inf  Measurements=off
  IGBT/Diode1 : spsIGBTDiodeLib/IGBT//Diode  Ron=1e-3  Rs=1e5  Cs=inf  Measurements=off
  Series RLC Branch : spsSeriesRLCBranchLib/Series RLC Branch  LConnTagsString=__new0  RConnTagsString=__new0  BranchType=RC  Resistance=0.01  Inductance=1e-3  SetiL0=off  InitialCurrent=0  Capacitance=500e-6  Setx0=on  InitialVoltage=Vdc  Measurements=None
  V : Terminator
  Voltage Measurement : spsVoltageMeasurementLib/Voltage Measurement  PhasorSimulation=off  OutputType=Complex  PSBequivalent=0
  DC+ : PMIOPort  Side=Left
  DC- : PMIOPort  Port=2  Side=Left
  AC : PMIOPort  Port=3  Side=Right
  I : Outport
  wires:
  s/1 -> Demux/1
  Current Measurement/1 -> I/1
  Voltage Measurement/1 -> V/1
  Demux/2 -> IGBT/Diode1/1
  Demux/1 -> IGBT/Diode/1
  connections:
  DC+/RConn1 -- Series RLC Branch/LConn1 -- Voltage Measurement/LConn1 -- IGBT/Diode/LConn1
  DC-/RConn1 -- Series RLC Branch/RConn1 -- Voltage Measurement/LConn2 -- IGBT/Diode1/RConn1
  IGBT/Diode/RConn1 -- Current Measurement/LConn1 -- IGBT/Diode1/LConn1
  AC/RConn1 -- Current Measurement/RConn1

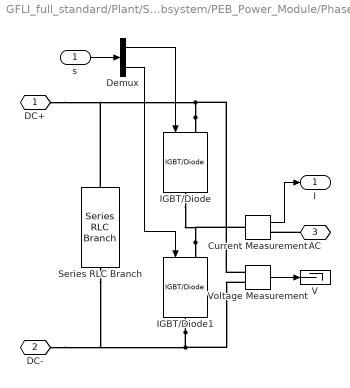
== system GFLI_full_standard/Plant/Subsystem/PEB_Power_Module/Phase B ==
  s : Inport
  Current Measurement : spsCurrentMeasurementLib/Current Measurement  PhasorSimulation=off  OutputType=Complex  PSBequivalent=0
  Demux : Demux  Outputs=2
  IGBT/Diode : spsIGBTDiodeLib/IGBT//Diode  Ron=1e-3  Rs=1e5  Cs=inf  Measurements=off
  IGBT/Diode1 : spsIGBTDiodeLib/IGBT//Diode  Ron=1e-3  Rs=1e5  Cs=inf  Measurements=off
  Series RLC Branch : spsSeriesRLCBranchLib/Series RLC Branch  LConnTagsString=__new0  RConnTagsString=__new0  BranchType=RC  Resistance=0.01  Inductance=1e-3  SetiL0=off  InitialCurrent=0  Capacitance=500e-6  Setx0=on  InitialVoltage=Vdc  Measurements=None
  V : Terminator
  Voltage Measurement : spsVoltageMeasurementLib/Voltage Measurement  PhasorSimulation=off  OutputType=Complex  PSBequivalent=0
  DC+ : PMIOPort  Side=Left
  DC- : PMIOPort  Port=2  Side=Left
  AC : PMIOPort  Port=3  Side=Right
  I : Outport
  wires:
  Demux/1 -> IGBT/Diode/1
  Demux/2 -> IGBT/Diode1/1
  Voltage Measurement/1 -> V/1
  Current Measurement/1 -> I/1
  s/1 -> Demux/1
  connections:
  AC/RConn1 -- Current Measurement/RConn1
  IGBT/Diode1/LConn1 -- Current Measurement/LConn1 -- IGBT/Diode/RConn1
  IGBT/Diode1/RConn1 -- Voltage Measurement/LConn2 -- Series RLC Branch/RConn1 -- DC-/RConn1
  IGBT/Diode/LConn1 -- Voltage Measurement/LConn1 -- Series RLC Branch/LConn1 -- DC+/RConn1

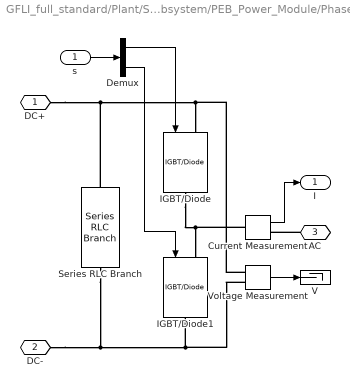
== system GFLI_full_standard/Plant/Subsystem/PEB_Power_Module/Phase C ==
  s : Inport
  Current Measurement : spsCurrentMeasurementLib/Current Measurement  PhasorSimulation=off  OutputType=Complex  PSBequivalent=0
  Demux : Demux  Outputs=2
  IGBT/Diode : spsIGBTDiodeLib/IGBT//Diode  Ron=1e-3  Rs=1e5  Cs=inf  Measurements=off
  IGBT/Diode1 : spsIGBTDiodeLib/IGBT//Diode  Ron=1e-3  Rs=1e5  Cs=inf  Measurements=off
  Series RLC Branch : spsSeriesRLCBranchLib/Series RLC Branch  LConnTagsString=__new0  RConnTagsString=__new0  BranchType=RC  Resistance=0.01  Inductance=1e-3  SetiL0=off  InitialCurrent=0  Capacitance=500e-6  Setx0=on  InitialVoltage=Vdc  Measurements=None
  V : Terminator
  Voltage Measurement : spsVoltageMeasurementLib/Voltage Measurement  PhasorSimulation=off  OutputType=Complex  PSBequivalent=0
  DC+ : PMIOPort  Side=Left
  DC- : PMIOPort  Port=2  Side=Left
  AC : PMIOPort  Port=3  Side=Right
  I : Outport
  wires:
  s/1 -> Demux/1
  Current Measurement/1 -> I/1
  Voltage Measurement/1 -> V/1
  Demux/2 -> IGBT/Diode1/1
  Demux/1 -> IGBT/Diode/1
  connections:
  DC+/RConn1 -- Series RLC Branch/LConn1 -- Voltage Measurement/LConn1 -- IGBT/Diode/LConn1
  DC-/RConn1 -- Series RLC Branch/RConn1 -- Voltage Measurement/LConn2 -- IGBT/Diode1/RConn1
  IGBT/Diode/RConn1 -- Current Measurement/LConn1 -- IGBT/Diode1/LConn1
  AC/RConn1 -- Current Measurement/RConn1
